simulink model "LoopSimulation"  (R2025a)
settings: Solver=VariableStepAuto  StartTime=0.0  StopTime=3  RelTol=1e-3
values from neighbouring files (symbols this model uses):
  capacitances = [capacitances.C_iss	capacitances.C_oss	capacitances.C_rss]    [simulink_variables.m]
undefined symbols (not defined in the file or in its folder): capacitance_vds, id, vds, vgs
libraries: simulink x9, cstblocks x7
settings Model: Creator=josephderay  LastModifiedBy=josephderay

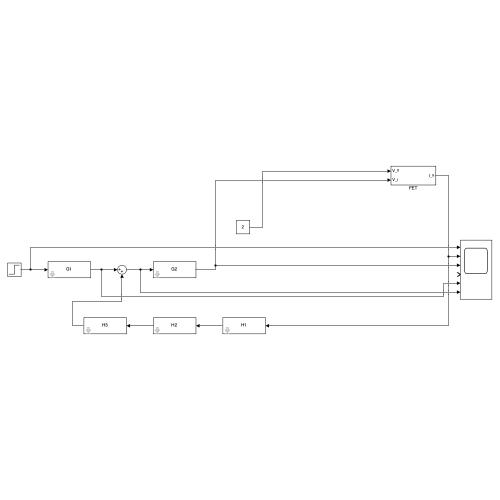
[thumbnail: Simulink's stored preview of the top-level diagram]
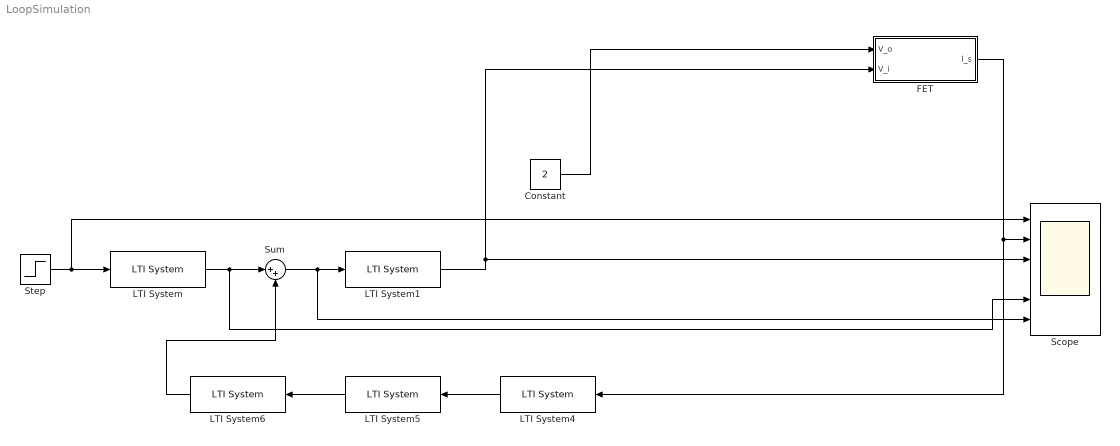
== system LoopSimulation ==
  Constant : Constant  Value=2
  FET : Subsystem
  LTI System : cstblocks/LTI System  sys=G1  IC=[]  PadeOrder=0
  LTI System1 : cstblocks/LTI System  sys=G2  IC=[]  PadeOrder=0
  LTI System4 : cstblocks/LTI System  sys=H1  IC=[]  PadeOrder=0
  LTI System5 : cstblocks/LTI System  sys=H2  IC=[]  PadeOrder=0
  LTI System6 : cstblocks/LTI System  sys=H3  IC=[]  PadeOrder=0
  Scope : Scope  NumInputPorts=6
      settings: ActiveDisplayYMinimum=-31.428952207951269  ActiveDisplayYMaximum=93.488819260585629
  Step : Step  SampleTime=0
  Sum : Sum  Inputs=|++
  wires:
  LTI System/1 -> Scope/5, Sum/1
  Step/1 -> Scope/1, LTI System/1
  LTI System6/1 -> Sum/2
  Sum/1 -> Scope/6, LTI System1/1
  Constant/1 -> FET/1(V_o)
  LTI System4/1 -> LTI System5/1
  LTI System5/1 -> LTI System6/1
  FET/1(I_s) -> LTI System4/1, Scope/2
  LTI System1/1 -> Scope/3, FET/2(V_i)

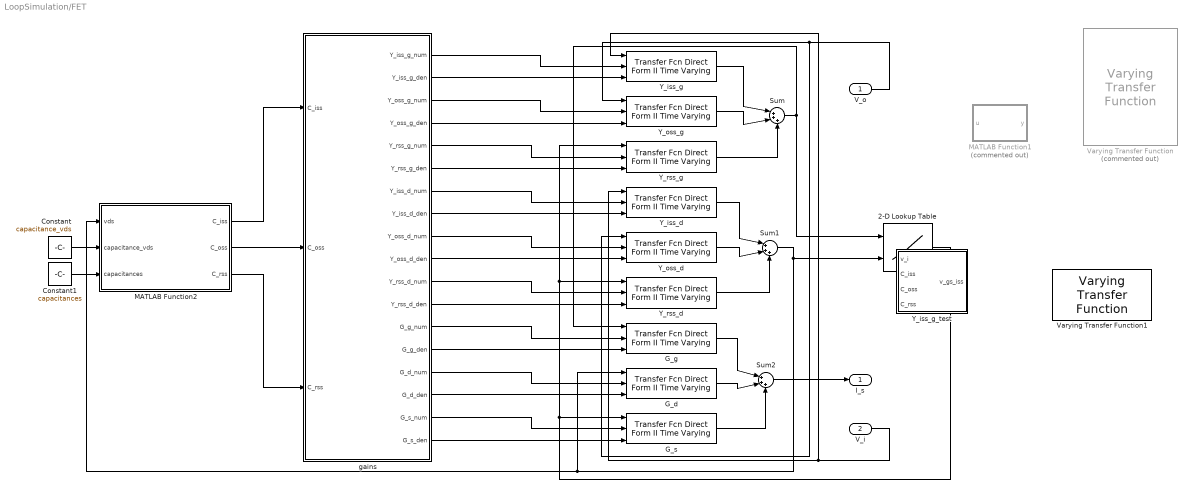
== system LoopSimulation/FET ==
  V_o : Inport
  V_i : Inport  Port=2
  2-D Lookup Table : Lookup_n-D  BreakpointsForDimension1=vgs  BreakpointsForDimension2=vds  Table=id  InternalRulePriority=Speed  RndMeth=Simplest
      settings: InputPortMap=u0,u1
  Constant : Constant  Value=capacitance_vds
  Constant1 : Constant  Value=capacitances
  G_d : simulink/Additional Math & Discrete/Additional Discrete/Transfer Fcn Direct Form II Time Varying  vinit=0.0  DoSatur=off
  G_g : simulink/Additional Math & Discrete/Additional Discrete/Transfer Fcn Direct Form II Time Varying  vinit=0.0  DoSatur=off
  G_s : simulink/Additional Math & Discrete/Additional Discrete/Transfer Fcn Direct Form II Time Varying  vinit=0.0  DoSatur=off
  MATLAB Function1 : MATLAB Function  Commented=on  TreatAsAtomicUnit=on
  MATLAB Function2 : MATLAB Function  TreatAsAtomicUnit=on
  Sum : Sum  Inputs=|+++
  Sum1 : Sum  Inputs=|+++
  Sum2 : Sum  Inputs=|+++
  Varying Transfer Function : cstblocks/Linear Parameter Varying/Varying Transfer Function  Commented=on  N=2  Feedthrough=on
  Varying Transfer Function1 : cstblocks/Linear Parameter Varying/Varying Transfer Function  N=1  Feedthrough=on
  Y_iss_d : simulink/Additional Math & Discrete/Additional Discrete/Transfer Fcn Direct Form II Time Varying  vinit=0.0  DoSatur=off
  Y_iss_g : simulink/Additional Math & Discrete/Additional Discrete/Transfer Fcn Direct Form II Time Varying  vinit=0.0  DoSatur=off
  Y_iss_g_test : Subsystem
  Y_oss_d : simulink/Additional Math & Discrete/Additional Discrete/Transfer Fcn Direct Form II Time Varying  vinit=0.0  DoSatur=off
  Y_oss_g : simulink/Additional Math & Discrete/Additional Discrete/Transfer Fcn Direct Form II Time Varying  vinit=0.0  DoSatur=off
  Y_rss_d : simulink/Additional Math & Discrete/Additional Discrete/Transfer Fcn Direct Form II Time Varying  vinit=0.0  DoSatur=off
  Y_rss_g : simulink/Additional Math & Discrete/Additional Discrete/Transfer Fcn Direct Form II Time Varying  vinit=0.0  DoSatur=off
  gains : MATLAB Function  TreatAsAtomicUnit=on
  I_s : Outport
  wires:
  gains/1(Y_iss_g_num) -> Y_iss_g/2
  gains/2(Y_iss_g_den) -> Y_iss_g/3
  gains/3(Y_oss_g_num) -> Y_oss_g/2
  gains/4(Y_oss_g_den) -> Y_oss_g/3
  gains/5(Y_rss_g_num) -> Y_rss_g/2
  gains/6(Y_rss_g_den) -> Y_rss_g/3
  gains/7(Y_iss_d_num) -> Y_iss_d/2
  gains/8(Y_iss_d_den) -> Y_iss_d/3
  gains/9(Y_oss_d_num) -> Y_oss_d/2
  gains/10(Y_oss_d_den) -> Y_oss_d/3
  gains/12(Y_rss_d_den) -> Y_rss_d/3
  gains/11(Y_rss_d_num) -> Y_rss_d/2
  gains/13(G_g_num) -> G_g/2
  gains/14(G_g_den) -> G_g/3
  gains/15(G_d_num) -> G_d/2
  gains/16(G_d_den) -> G_d/3
  gains/17(G_s_num) -> G_s/2
  gains/18(G_s_den) -> G_s/3
  V_i/1 -> Y_iss_g/1, Y_iss_d/1
  V_o/1 -> Y_oss_d/1, Y_oss_g/1
  2-D Lookup Table/1 -> G_s/1, Y_rss_d/1, Y_rss_g/1
  Y_iss_g/1 -> Sum/1
  Y_oss_g/1 -> Sum/2
  Y_rss_g/1 -> Sum/3
  Y_iss_d/1 -> Sum1/1
  Y_oss_d/1 -> Sum1/2
  Y_rss_d/1 -> Sum1/3
  G_g/1 -> Sum2/1
  G_d/1 -> Sum2/2
  G_s/1 -> Sum2/3
  Sum/1 -> 2-D Lookup Table/1, G_g/1
  Sum1/1 -> G_d/1, MATLAB Function2/1(vds), 2-D Lookup Table/2
  Sum2/1 -> I_s/1
  Constant1/1 -> MATLAB Function2/3(capacitances)
  Constant/1 -> MATLAB Function2/2(capacitance_vds)
  MATLAB Function2/1(C_iss) -> gains/1(C_iss)
  MATLAB Function2/2(C_oss) -> gains/2(C_oss)
  MATLAB Function2/3(C_rss) -> gains/3(C_rss)

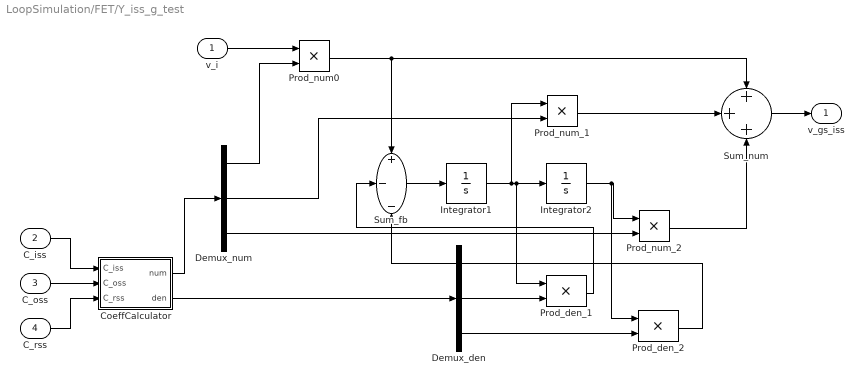
== system LoopSimulation/FET/Y_iss_g_test ==
  v_i : Inport
  C_iss : Inport  Port=2
  C_oss : Inport  Port=3
  C_rss : Inport  Port=4
  CoeffCalculator : MATLAB Function  TreatAsAtomicUnit=on
  Demux_den : Demux  Outputs=3
  Demux_num : Demux  Outputs=3
  Integrator1 : Integrator
  Integrator2 : Integrator
  Prod_den_1 : Product
  Prod_den_2 : Product
  Prod_num0 : Product
  Prod_num_1 : Product
  Prod_num_2 : Product
  Sum_fb : Sum  Inputs=+--
  Sum_num : Sum  Inputs=+++
  v_gs_iss : Outport
  wires:
  Sum_num/1 -> v_gs_iss/1
  Prod_den_2/1 -> Sum_fb/3
  Integrator2/1 -> Prod_num_2/1, Prod_den_2/1
  Demux_den/3 -> Prod_den_2/2
  Sum_fb/1 -> Integrator1/1
  Prod_num_1/1 -> Sum_num/2
  Demux_num/3 -> Prod_num_2/2
  Demux_den/2 -> Prod_den_1/2
  C_rss/1 -> CoeffCalculator/3(C_rss)
  Demux_num/1 -> Prod_num0/2
  v_i/1 -> Prod_num0/1
  CoeffCalculator/2(den) -> Demux_den/1
  Integrator1/1 -> Integrator2/1, Prod_den_1/1, Prod_num_1/1
  Prod_num0/1 -> Sum_num/1, Sum_fb/1
  Prod_num_2/1 -> Sum_num/3
  C_oss/1 -> CoeffCalculator/2(C_oss)
  Demux_num/2 -> Prod_num_1/2
  Prod_den_1/1 -> Sum_fb/2
  CoeffCalculator/1(num) -> Demux_num/1
  C_iss/1 -> CoeffCalculator/1(C_iss)

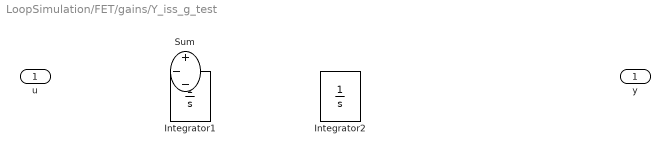
== system LoopSimulation/FET/gains/Y_iss_g_test ==
  u : Inport
  Integrator1 : Integrator
  Integrator2 : Integrator
  Sum : Sum  Inputs=+--
  y : Outport

== matlab function LoopSimulation/FET/Y_iss_g_test/CoeffCalculator ==
  data: C_iss input; num output; C_oss input; C_rss input; den output
function [num,den] = CoeffCalculator(C_iss,C_oss,C_rss)
%#codegen

%    This function was generated by the Symbolic Math Toolbox version 25.1.
%    30-Jul-2025 11:48:15

% C_iss = complex(C_iss);  % if required to enforce complex operations
% C_oss = complex(C_oss);  % if required to enforce complex operations
% C_rss = complex(C_rss);  % if required to enforce complex operations
t2 = C_rss.^2;
t3 = C_iss.*C_oss.*5.0e+9;
t4 = -t3;
t5 = t2.*5.0e+9;
t6 = t4+t5;
t7 = 1.0./t6;
t8 = t7.*2.00000001e+8;
t9 = -t8;
num = [0.0,C_oss.*t7.*-1.0e+9,t9];
if nargout > 1
    den = [1.0,-t7.*(C_iss.*1.000000005e+9+C_oss.*1.0e+9),t9];
end
end

== matlab function LoopSimulation/FET/MATLAB Function1 ==
  data: u input; y output
function y = fcn(u)
[g_m, r_o] = drain_curves(0);
y = u;

== matlab function LoopSimulation/FET/MATLAB Function2 ==
  data: vds input; C_iss output; C_oss output; C_rss output; capacitance_vds input; capacitances input
function [C_iss, C_oss, C_rss] = capacitances(vds, capacitance_vds, capacitances)
    values = interp1(capacitance_vds, capacitances, vds);
    C_iss = values(:, 1);
    C_oss = values(:, 2);
    C_rss = values(:, 3);
end

== matlab function LoopSimulation/FET/gains ==
  data: C_iss input; Y_iss_g_num output; C_oss input; C_rss input; Y_iss_g_den output; Y_oss_g_num output; Y_oss_g_den output; Y_rss_g_num output; Y_rss_g_den output; Y_iss_d_num output; Y_iss_d_den output; Y_oss_d_num output; Y_oss_d_den output; Y_rss_d_num output; Y_rss_d_den output; G_g_num output; G_g_den output; G_d_num output; G_d_den output; G_s_num output; G_s_den output
function [Y_iss_g_num,Y_iss_g_den,Y_oss_g_num,Y_oss_g_den,Y_rss_g_num,Y_rss_g_den,Y_iss_d_num,Y_iss_d_den,Y_oss_d_num,Y_oss_d_den,Y_rss_d_num,Y_rss_d_den,G_g_num,G_g_den,G_d_num,G_d_den,G_s_num,G_s_den] = gains(C_iss,C_oss,C_rss)
%#codegen

%    This function was generated by the Symbolic Math Toolbox version 25.1.
%    29-Jul-2025 10:40:49

% C_iss = complex(C_iss);  % if required to enforce complex operations
% C_oss = complex(C_oss);  % if required to enforce complex operations
% C_rss = complex(C_rss);  % if required to enforce complex operations
t2 = C_rss.^2;
t3 = C_iss.*C_oss;
t4 = -C_rss;
t11 = C_iss.*2.00000001e+8;
t12 = C_oss.*2.0e+8;
t5 = t3.*5.0;
t6 = t2.*5.0;
t7 = -t3;
t17 = t11+t12;
t9 = t2+t7;
t14 = -1.0./(t5-t6);
t13 = 1.0./t9;
t16 = t4.*t14;
t18 = t13.*4.00000002e-2;
t20 = (t13.*t17)./1.0e+9;
t19 = -t18;
Y_iss_g_num = [C_oss./(t5-t6),t19];
if nargout > 1
    t21 = -t20;
    Y_iss_g_den = [t21,t19];
end
if nargout > 2
    Y_oss_g_num = [t16,0.0];
end
if nargout > 3
    Y_oss_g_den = [t21,t19];
end
if nargout > 4
    Y_rss_g_num = [C_rss.*t13,0.0];
end
if nargout > 5
    Y_rss_g_den = [t21,t19];
end
if nargout > 6
    Y_iss_d_num = [t16,0.0];
end
if nargout > 7
    Y_iss_d_den = [t21,t19];
end
if nargout > 8
    Y_oss_d_num = [C_iss./(t5-t6),-1.0./(t2.*2.5e+1-t3.*2.5e+1)];
end
if nargout > 9
    Y_oss_d_den = [t21,t19];
end
if nargout > 10
    Y_rss_d_num = [C_iss.*t13,t14];
end
if nargout > 11
    Y_rss_d_den = [t21,t19];
end
if nargout > 12
    G_g_num = [C_iss+t4,0.0,0.0];
end
if nargout > 13
    G_g_den = 0.0;
end
if nargout > 14
    G_d_num = [C_oss+t4,1.0e-9,0.0];
end
if nargout > 15
    G_d_den = 0.0;
end
if nargout > 16
    G_s_num = [1.0,0.0];
end
if nargout > 17
    G_s_den = 0.0;
end
end
